simulink model "Variable_spring_CBF_Liu"  (R2023b)
settings: Solver=ode5  StartTime=0.0  StopTime=4  FixedStep=0.0001  RelTol=1e-3
settings Model: Creator=amaiani  LastModifiedBy=amaiani

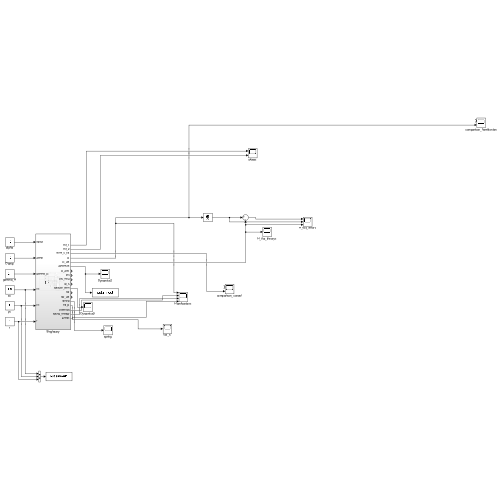
[thumbnail: Simulink's stored preview of the top-level diagram]
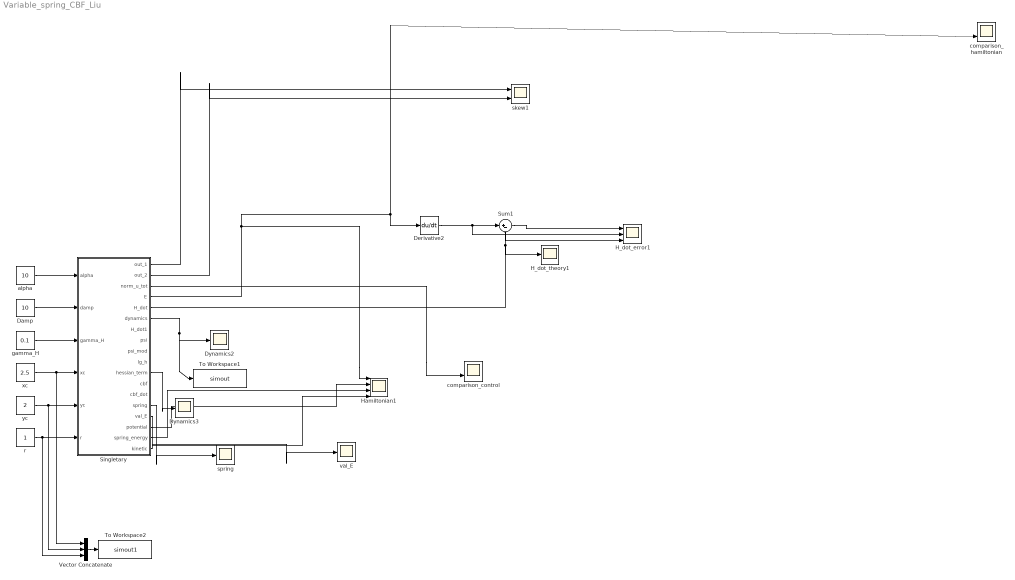
== system Variable_spring_CBF_Liu ==
  Damp : Constant  Value=10
  Derivative2 : Derivative
  Dynamics2 : Scope
  Dynamics3 : Scope
  H_dot_error1 : Scope  NumInputPorts=3
  H_dot_theory1 : Scope
  Hamiltonian1 : Scope  NumInputPorts=4
  Singletary : Subsystem
  Sum1 : Sum  Inputs=|+-
  To Workspace1 : ToWorkspace  VariableName=simout  SampleTime=-1
  To Workspace2 : ToWorkspace  VariableName=simout1  SampleTime=-1
  Vector Concatenate : Concatenate  NumInputs=3
  alpha : Constant  Value=10
  comparison_control : Scope  NumInputPorts=2
  comparison_hamiltonian : Scope  NumInputPorts=2
  gamma_H : Constant  Value=0.1
  r : Constant
  skew1 : Scope  NumInputPorts=2
  spring : Scope
  val_E : Scope
  xc : Constant  Value=2.5
  yc : Constant  Value=2
  wires:
  Derivative2/1 -> H_dot_error1/2, Sum1/1
  Damp/1 -> Singletary/2(damp)
  Sum1/1 -> H_dot_error1/1
  alpha/1 -> Singletary/1(alpha)
  Singletary/5(H_dot) -> H_dot_theory1/1, H_dot_error1/3, Sum1/2
  Singletary/4(E) -> Derivative2/1, comparison_hamiltonian/2, Hamiltonian1/1
  Singletary/1(out_1) -> skew1/1
  Singletary/2(out_2) -> skew1/2
  Singletary/3(norm_u_tot) -> comparison_control/2
  Singletary/6(dynamics) -> Dynamics2/1, To Workspace1/1
  Singletary/11(hessian_term) -> Dynamics3/1
  Singletary/14(spring) -> spring/1
  Singletary/15(val_E) -> val_E/1
  Singletary/18(kinetic) -> Hamiltonian1/4
  Singletary/17(spring_energy) -> Hamiltonian1/3
  Singletary/16(potential) -> Hamiltonian1/2
  gamma_H/1 -> Singletary/3(gamma_H)
  xc/1 -> Vector Concatenate/1, Singletary/4(xc)
  yc/1 -> Vector Concatenate/2, Singletary/5(yc)
  r/1 -> Vector Concatenate/3, Singletary/6(r)
  Vector Concatenate/1 -> To Workspace2/1

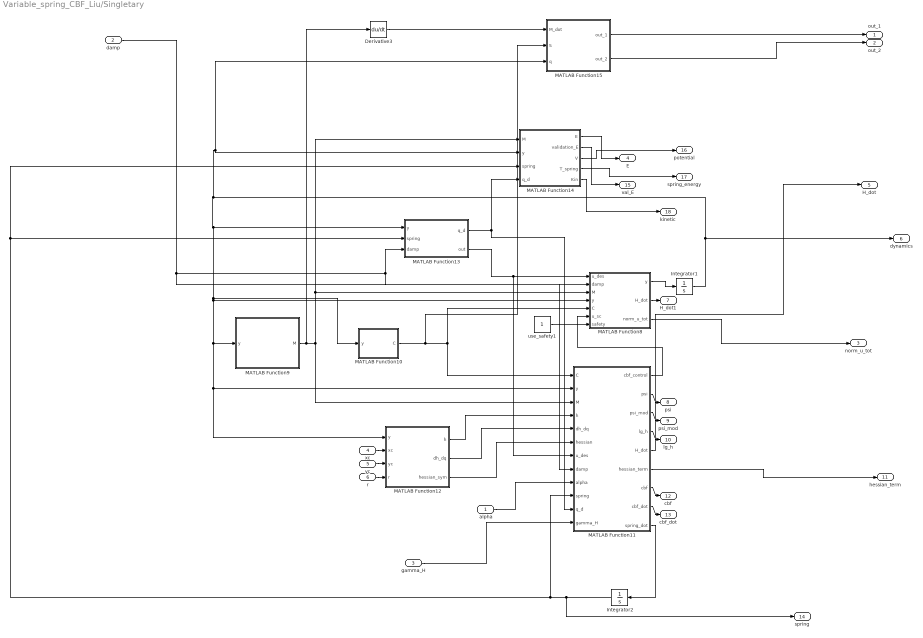
== system Variable_spring_CBF_Liu/Singletary ==
  alpha : Inport
  damp : Inport  Port=2
  gamma_H : Inport  Port=3
  xc : Inport  Port=4
  yc : Inport  Port=5
  r : Inport  Port=6
  Derivative3 : Derivative
  Integrator1 : Integrator  InitialCondition=[0;0;0;0;0;0]
  Integrator2 : Integrator  InitialCondition=[10;10;10]
  MATLAB Function10 : MATLAB Function  StartFcn=|  TreatAsAtomicUnit=on
      | % Define numerical values for the parameters
      | xc = 2.5;
      | yc = 2;
      | r = 1;
      | gamma = 2;
      | alpha = 20;
      | 
      | 
      | m1 = 1;
      | m2 = 1;
      | m3 = 1;
      | 
      | 
      | l1 = 1;
      | l2 = 1;
      | l3 = 1;
  MATLAB Function11 : MATLAB Function  TreatAsAtomicUnit=on
  MATLAB Function12 : MATLAB Function  TreatAsAtomicUnit=on
  MATLAB Function13 : MATLAB Function  TreatAsAtomicUnit=on
  MATLAB Function14 : MATLAB Function  TreatAsAtomicUnit=on
  MATLAB Function15 : MATLAB Function  StartFcn=|  TreatAsAtomicUnit=on
      | % Define numerical values for the parameters
      | xc = 2.5;
      | yc = 2;
      | r = 1;
      | gamma = 2;
      | alpha = 20;
      | 
      | 
      | m1 = 1;
      | m2 = 1;
      | m3 = 1;
      | 
      | 
      | l1 = 1;
      | l2 = 1;
      | l3 = 1;
  MATLAB Function8 : MATLAB Function  TreatAsAtomicUnit=on
  MATLAB Function9 : MATLAB Function  StartFcn=|  TreatAsAtomicUnit=on
      | % Define numerical values for the parameters
      | xc = 2.5;
      | yc = 2;
      | r = 1;
      | gamma = 2;
      | alpha = 20;
      | 
      | 
      | m1 = 1;
      | m2 = 1;
      | m3 = 1;
      | 
      | 
      | l1 = 1;
      | l2 = 1;
      | l3 = 1;
  use_safety1 : Constant
  out_1 : Outport
  out_2 : Outport  Port=2
  norm_u_tot : Outport  Port=3
  E : Outport  Port=4
  H_dot : Outport  Port=5
  dynamics : Outport  Port=6
  H_dot1 : Outport  Port=7
  psi : Outport  Port=8
  psi_mod : Outport  Port=9
  lg_h : Outport  Port=10
  hessian_term : Outport  Port=11
  cbf : Outport  Port=12
  cbf_dot : Outport  Port=13
  spring : Outport  Port=14
  val_E : Outport  Port=15
  potential : Outport  Port=16
  spring_energy : Outport  Port=17
  kinetic : Outport  Port=18
  wires:
  MATLAB Function11/2(psi) -> psi/1
  MATLAB Function11/4(lg_h) -> lg_h/1
  MATLAB Function11/7(cbf) -> cbf/1
  MATLAB Function8/2(H_dot) -> H_dot1/1
  MATLAB Function11/5(H_dot) -> H_dot/1
  MATLAB Function11/6(hessian_term) -> hessian_term/1
  MATLAB Function14/1(E) -> E/1
  MATLAB Function8/3(norm_u_tot) -> norm_u_tot/1
  MATLAB Function12/3(hessian_sym) -> MATLAB Function11/6(hessian)
  Derivative3/1 -> MATLAB Function15/1(M_dot)
  MATLAB Function12/1(h) -> MATLAB Function11/4(h)
  MATLAB Function8/1(y) -> Integrator1/1
  MATLAB Function11/3(psi_mod) -> psi_mod/1
  alpha/1 -> MATLAB Function11/9(alpha)
  MATLAB Function10/1(C) -> MATLAB Function8/5(C), MATLAB Function11/1(C), MATLAB Function15/2(S)
  MATLAB Function11/1(cbf_control) -> MATLAB Function8/6(u_sc)
  MATLAB Function15/2(out_2) -> out_2/1
  Integrator1/1 -> dynamics/1, MATLAB Function15/3(q), MATLAB Function14/2(y), MATLAB Function13/1(y), MATLAB Function10/1(y), MATLAB Function12/1(y), MATLAB Function11/2(y), MATLAB Function9/1(y), MATLAB Function8/4("y ")
  MATLAB Function15/1(out_1) -> out_1/1
  damp/1 -> MATLAB Function11/8(damp), MATLAB Function8/2(damp), MATLAB Function13/3(damp)
  MATLAB Function12/2(dh_dq) -> MATLAB Function11/5(dh_dq)
  MATLAB Function13/2(out) -> MATLAB Function11/7(u_des), MATLAB Function8/1(u_des)
  MATLAB Function11/8(cbf_dot) -> cbf_dot/1
  use_safety1/1 -> MATLAB Function8/7(safety)
  MATLAB Function9/1(M) -> Derivative3/1, MATLAB Function14/1(M), MATLAB Function8/3(M), MATLAB Function11/3(M)
  MATLAB Function11/9(spring_dot) -> Integrator2/1
  Integrator2/1 -> spring/1, MATLAB Function11/10(spring), MATLAB Function13/2(spring), MATLAB Function14/3(spring)
  MATLAB Function13/1(q_d) -> MATLAB Function11/11(q_d), MATLAB Function14/4(q_d)
  MATLAB Function14/2(validation_E) -> val_E/1
  MATLAB Function14/3(V) -> potential/1
  MATLAB Function14/4(T_spring) -> spring_energy/1
  MATLAB Function14/5(Kin) -> kinetic/1
  gamma_H/1 -> MATLAB Function11/12(gamma_H)
  xc/1 -> MATLAB Function12/2(xc)
  yc/1 -> MATLAB Function12/3(yc)
  r/1 -> MATLAB Function12/4(r)

== matlab function Variable_spring_CBF_Liu/Singletary/MATLAB Function8 ==
  data: u_des input; damp input; M input; y input; y output; C input; H_dot output; u_sc input; safety input; norm_u_tot output
function [y,H_dot,norm_u_tot]= dynamics(u_des, damp , M,y, C, u_sc, safety)
    
    q = reshape(y(1:3),[3,1]);
    dq = reshape(y(4:6),[3,1]);



    [~, p] = chol(M);
    decision = (p == 0);

    assert(decision, 'Inertia matrix is not positive definite');
    
    u_tot = u_des + safety * u_sc;
    norm_u_tot=norm(u_tot);
    ddq = inv(M) * (u_tot - C * dq ); % + u_sc

    H_dot = - dq' * damp * dq;

    y = [dq; ddq];

== matlab function Variable_spring_CBF_Liu/Singletary/MATLAB Function9 ==
  data: y input; M output
function M = inertia_M(y)

    q1 = y(1);
    q2 = y(2);
    q3 = y(3);

    M  = [        cos(q2 + q3) + 3*cos(q2) + cos(q3) + 4, cos(q2 + q3)/2 + (3*cos(q2))/2 + cos(q3) + 5/3, cos(q2 + q3)/2 + cos(q3)/2 + 1/3;
cos(q2 + q3)/2 + (3*cos(q2))/2 + cos(q3) + 5/3,                                  cos(q3) + 5/3,                  cos(q3)/2 + 1/3;
              cos(q2 + q3)/2 + cos(q3)/2 + 1/3,                                cos(q3)/2 + 1/3,                              1/3];

== matlab function Variable_spring_CBF_Liu/Singletary/MATLAB Function10 ==
  data: y input; C output
function C = coriolis(y)

    q1 = y(1);
    q2 = y(2);
    q3 = y(3);
    dq1 = y(4);
    dq2 = y(5);
    dq3 = y(6);


    C = [- dq2*(sin(q2 + q3)/2 + (3*sin(q2))/2) - dq3*(sin(q2 + q3)/2 + sin(q3)/2), - dq1*(sin(q2 + q3)/2 + (3*sin(q2))/2) - dq2*(sin(q2 + q3)/2 + (3*sin(q2))/2) - dq3*(sin(q2 + q3)/2 + sin(q3)/2), - dq1*(sin(q2 + q3)/2 + sin(q3)/2) - dq2*(sin(q2 + q3)/2 + sin(q3)/2) - dq3*(sin(q2 + q3)/2 + sin(q3)/2);
                dq1*(sin(q2 + q3)/2 + (3*sin(q2))/2) - (dq3*sin(q3))/2,                                                                                                 -(dq3*sin(q3))/2,                                                    - (dq1*sin(q3))/2 - (dq2*sin(q3))/2 - (dq3*sin(q3))/2;
                       dq1*(sin(q2 + q3)/2 + sin(q3)/2) + (dq2*sin(q3))/2,                                                                                (dq1*sin(q3))/2 + (dq2*sin(q3))/2,                                                                                                        0];

== matlab function Variable_spring_CBF_Liu/Singletary/MATLAB Function11 ==
  data: C input; y input; cbf_control output; M input; h input; dh_dq input; hessian input; u_des input; psi output; psi_mod output; lg_h output; H_dot output; damp input; hessian_term output; cbf output; cbf_dot output; alpha input; spring_dot output; spring input; q_d input; gamma_H input

function [cbf_control, psi, psi_mod,lg_h, H_dot, hessian_term, cbf, cbf_dot, spring_dot]= CBF(C, y, M, h, dh_dq, hessian, u_des, damp, alpha, spring, q_d, gamma_H)
% Define numerical values for the parameters
    xc = 2.5;
    yc = 2;
    r = 1;
    gamma = 2;

    
    m1 = 1;
    m2 = 1;
    m3 = 1;
    
    l1 = 1;
    l2 = 1;
    l3 = 1;
    
    q = reshape(y(1:3),[3,1]);
    dq = reshape(y(4:6),[3,1]);
    dh_dq = reshape(dh_dq,[1,3]);


    cbf = alpha * h + dh_dq * dq;
    lg_h = zeros(1,3);

    M_inv = inv(M);
    cbf_dot_prior = alpha .* dh_dq * dq + dq' * hessian * dq + dh_dq * (M_inv* (-C * dq + u_des));
    psi = cbf_dot_prior + gamma .* cbf;
    if psi<0
        lg_h = dh_dq * M_inv;
        
        cbf_control =  - lg_h' /(lg_h * lg_h')  .* psi;
        active = 1;
    else
        cbf_control = zeros(3,1);

    end
    cbf_dot = alpha .* dh_dq * dq + dq' * hessian * dq + dh_dq * M_inv* (-C * dq + u_des+ cbf_control);
    psi_mod = cbf_dot + gamma .* cbf;

    
    
    dissipated= - dq' * damp * dq;

    hessian_term = dq' * hessian * dq;
    
    spring_dot = zeros(3,1);


    H_dot = dq' * cbf_control - dq' * damp * dq + gamma_H * (0.5 * dq' * M * dq + 0.5 * (q-q_d)' * diag(spring) * (q-q_d) + 0.5 * spring' * spring);
    if psi<0
        error_term = 0.5 * (q-q_d) .* (q-q_d);
        
        A_matrix = error_term' + spring';
    
        spring_dot = -A_matrix'/norm(A_matrix')^2*H_dot;
    
        spring_min = 1;
        gamma_spring = 5;
        spring_dot_min=-gamma_spring * (spring-spring_min);
        spring_dot = max(spring_dot,spring_dot_min);
        spring_dot = min(spring_dot,10 * ones(3,1));
        H_dot = H_dot + A_matrix * spring_dot;
    else

        spring_dot = zeros(3,1);
    end
    
end

== matlab function Variable_spring_CBF_Liu/Singletary/MATLAB Function12 ==
  data: y input; h output; dh_dq output; hessian_sym output; xc input; yc input; r input
function [h, dh_dq, hessian_sym] = obstacle(y,xc,yc,r)
    % Define numerical values for the parameters
    % xc = -2.5;
    % yc = 2;
    % r = 1;

    l1 = 1;
    l2 = 1;
    l3 = 1;
    
    % Compute the end-effector position using forward kinematics
    q1 = y(1);
    q2 = y(2);
    q3 = y(3);
    
    x_ee = l1 * cos(q1) + l2 * cos(q1 + q2) + l3 * cos(q1 + q2 + q3);
    y_ee = l1 * sin(q1) + l2 * sin(q1 + q2) + l3 * sin(q1 + q2 + q3);
    
    % Compute the control barrier function h
    h = (xc - x_ee)^2 + (yc - y_ee)^2 - r^2;
    
    % Define the expressions for dh_dq and hessian_sym
    % dh_dq = [2*(cos(q1 + q2 + q3) + cos(q1 + q2) + cos(q1))*(sin(q1 + q2 + q3) + sin(q1 + q2) + sin(q1) - 2) - 2*(sin(q1 + q2 + q3) + sin(q1 + q2) + sin(q1))*(cos(q1 + q2 + q3) + cos(q1 + q2) + cos(q1) - 5/2), 2*(cos(q1 + q2 + q3) + cos(q1 + q2))*(sin(q1 + q2 + q3) + sin(q1 + q2) + sin(q1) - 2) - 2*(sin(q1 + q2 + q3) + sin(q1 + q2))*(cos(q1 + q2 + q3) + cos(q1 + q2) + cos(q1) - 5/2), 2*cos(q1 + q2 + q3)*(sin(q1 + q2 + q3) + sin(q1 + q2) + sin(q1) - 2) - 2*sin(q1 + q2 + q3)*(cos(q1 + q2 + q3) + cos(q1 + q2) + cos(q1) - 5/2)];
    dh_dq = [2*(cos(q1 + q2 + q3) + cos(q1 + q2) + cos(q1))*(sin(q1 + q2 + q3) - yc + sin(q1 + q2) + sin(q1)) - 2*(sin(q1 + q2 + q3) + sin(q1 + q2) + sin(q1))*(cos(q1 + q2 + q3) - xc + cos(q1 + q2) + cos(q1)), 2*(cos(q1 + q2 + q3) + cos(q1 + q2))*(sin(q1 + q2 + q3) - yc + sin(q1 + q2) + sin(q1)) - 2*(sin(q1 + q2 + q3) + sin(q1 + q2))*(cos(q1 + q2 + q3) - xc + cos(q1 + q2) + cos(q1)), 2*cos(q1 + q2 + q3)*(sin(q1 + q2 + q3) - yc + sin(q1 + q2) + sin(q1)) - 2*sin(q1 + q2 + q3)*(cos(q1 + q2 + q3) - xc + cos(q1 + q2) + cos(q1))];
 

    % hessian_sym = [                                              2*(cos(q1 + q2 + q3) + cos(q1 + q2) + cos(q1))^2 - 2*(cos(q1 + q2 + q3) + cos(q1 + q2) + cos(q1))*(cos(q1 + q2 + q3) + cos(q1 + q2) + cos(q1) - 5/2) + 2*(sin(q1 + q2 + q3) + sin(q1 + q2) + sin(q1))^2 - 2*(sin(q1 + q2 + q3) + sin(q1 + q2) + sin(q1))*(sin(q1 + q2 + q3) + sin(q1 + q2) + sin(q1) - 2), 2*(cos(q1 + q2 + q3) + cos(q1 + q2))*(cos(q1 + q2 + q3) + cos(q1 + q2) + cos(q1)) - 2*(cos(q1 + q2 + q3) + cos(q1 + q2))*(cos(q1 + q2 + q3) + cos(q1 + q2) + cos(q1) - 5/2) + 2*(sin(q1 + q2 + q3) + sin(q1 + q2))*(sin(q1 + q2 + q3) + sin(q1 + q2) + sin(q1)) - 2*(sin(q1 + q2 + q3) + sin(q1 + q2))*(sin(q1 + q2 + q3) + sin(q1 + q2) + sin(q1) - 2), 2*cos(q1 + q2 + q3)*(cos(q1 + q2 + q3) + cos(q1 + q2) + cos(q1)) - 2*cos(q1 + q2 + q3)*(cos(q1 + q2 + q3) + cos(q1 + q2) + cos(q1) - 5/2) + 2*sin(q1 + q2 + q3)*(sin(q1 + q2 + q3) + sin(q1 + q2) + sin(q1)) - 2*sin(q1 + q2 + q3)*(sin(q1 + q2 + q3) + sin(q1 + q2) + sin(q1) - 2);
    %     2*(cos(q1 + q2 + q3) + cos(q1 + q2))*(cos(q1 + q2 + q3) + cos(q1 + q2) + cos(q1)) - 2*(cos(q1 + q2 + q3) + cos(q1 + q2))*(cos(q1 + q2 + q3) + cos(q1 + q2) + cos(q1) - 5/2) + 2*(sin(q1 + q2 + q3) + sin(q1 + q2))*(sin(q1 + q2 + q3) + sin(q1 + q2) + sin(q1)) - 2*(sin(q1 + q2 + q3) + sin(q1 + q2))*(sin(q1 + q2 + q3) + sin(q1 + q2) + sin(q1) - 2),                                                                                       2*(cos(q1 + q2 + q3) + cos(q1 + q2))^2 - 2*(cos(q1 + q2 + q3) + cos(q1 + q2))*(cos(q1 + q2 + q3) + cos(q1 + q2) + cos(q1) - 5/2) + 2*(sin(q1 + q2 + q3) + sin(q1 + q2))^2 - 2*(sin(q1 + q2 + q3) + sin(q1 + q2))*(sin(q1 + q2 + q3) + sin(q1 + q2) + sin(q1) - 2),                     2*cos(q1 + q2 + q3)*(cos(q1 + q2 + q3) + cos(q1 + q2)) - 2*cos(q1 + q2 + q3)*(cos(q1 + q2 + q3) + cos(q1 + q2) + cos(q1) - 5/2) - 2*sin(q1 + q2 + q3)*(sin(q1 + q2 + q3) + sin(q1 + q2) + sin(q1) - 2) + 2*sin(q1 + q2 + q3)*(sin(q1 + q2 + q3) + sin(q1 + q2));
    %                                                                         2*cos(q1 + q2 + q3)*(cos(q1 + q2 + q3) + cos(q1 + q2) + cos(q1)) - 2*cos(q1 + q2 + q3)*(cos(q1 + q2 + q3) + cos(q1 + q2) + cos(q1) - 5/2) + 2*sin(q1 + q2 + q3)*(sin(q1 + q2 + q3) + sin(q1 + q2) + sin(q1)) - 2*sin(q1 + q2 + q3)*(sin(q1 + q2 + q3) + sin(q1 + q2) + sin(q1) - 2),                                                                                         2*cos(q1 + q2 + q3)*(cos(q1 + q2 + q3) + cos(q1 + q2)) - 2*cos(q1 + q2 + q3)*(cos(q1 + q2 + q3) + cos(q1 + q2) + cos(q1) - 5/2) - 2*sin(q1 + q2 + q3)*(sin(q1 + q2 + q3) + sin(q1 + q2) + sin(q1) - 2) + 2*sin(q1 + q2 + q3)*(sin(q1 + q2 + q3) + sin(q1 + q2)),                                                                                       2*cos(q1 + q2 + q3)^2 - 2*cos(q1 + q2 + q3)*(cos(q1 + q2 + q3) + cos(q1 + q2) + cos(q1) - 5/2) + 2*sin(q1 + q2 + q3)^2 - 2*sin(q1 + q2 + q3)*(sin(q1 + q2 + q3) + sin(q1 + q2) + sin(q1) - 2)];
    % 
    % 
    hessian_sym =    [                                              2*(cos(q1 + q2 + q3) + cos(q1 + q2) + cos(q1))^2 - 2*(cos(q1 + q2 + q3) + cos(q1 + q2) + cos(q1))*(cos(q1 + q2 + q3) - xc + cos(q1 + q2) + cos(q1)) - 2*(sin(q1 + q2 + q3) + sin(q1 + q2) + sin(q1))*(sin(q1 + q2 + q3) - yc + sin(q1 + q2) + sin(q1)) + 2*(sin(q1 + q2 + q3) + sin(q1 + q2) + sin(q1))^2, 2*(cos(q1 + q2 + q3) + cos(q1 + q2))*(cos(q1 + q2 + q3) + cos(q1 + q2) + cos(q1)) - 2*(cos(q1 + q2 + q3) + cos(q1 + q2))*(cos(q1 + q2 + q3) - xc + cos(q1 + q2) + cos(q1)) - 2*(sin(q1 + q2 + q3) + sin(q1 + q2))*(sin(q1 + q2 + q3) - yc + sin(q1 + q2) + sin(q1)) + 2*(sin(q1 + q2 + q3) + sin(q1 + q2))*(sin(q1 + q2 + q3) + sin(q1 + q2) + sin(q1)), 2*cos(q1 + q2 + q3)*(cos(q1 + q2 + q3) + cos(q1 + q2) + cos(q1)) - 2*cos(q1 + q2 + q3)*(cos(q1 + q2 + q3) - xc + cos(q1 + q2) + cos(q1)) - 2*sin(q1 + q2 + q3)*(sin(q1 + q2 + q3) - yc + sin(q1 + q2) + sin(q1)) + 2*sin(q1 + q2 + q3)*(sin(q1 + q2 + q3) + sin(q1 + q2) + sin(q1));
        2*(cos(q1 + q2 + q3) + cos(q1 + q2))*(cos(q1 + q2 + q3) + cos(q1 + q2) + cos(q1)) - 2*(cos(q1 + q2 + q3) + cos(q1 + q2))*(cos(q1 + q2 + q3) - xc + cos(q1 + q2) + cos(q1)) - 2*(sin(q1 + q2 + q3) + sin(q1 + q2))*(sin(q1 + q2 + q3) - yc + sin(q1 + q2) + sin(q1)) + 2*(sin(q1 + q2 + q3) + sin(q1 + q2))*(sin(q1 + q2 + q3) + sin(q1 + q2) + sin(q1)),                                                                                       2*(cos(q1 + q2 + q3) + cos(q1 + q2))^2 - 2*(cos(q1 + q2 + q3) + cos(q1 + q2))*(cos(q1 + q2 + q3) - xc + cos(q1 + q2) + cos(q1)) - 2*(sin(q1 + q2 + q3) + sin(q1 + q2))*(sin(q1 + q2 + q3) - yc + sin(q1 + q2) + sin(q1)) + 2*(sin(q1 + q2 + q3) + sin(q1 + q2))^2,                     2*cos(q1 + q2 + q3)*(cos(q1 + q2 + q3) + cos(q1 + q2)) - 2*sin(q1 + q2 + q3)*(sin(q1 + q2 + q3) - yc + sin(q1 + q2) + sin(q1)) - 2*cos(q1 + q2 + q3)*(cos(q1 + q2 + q3) - xc + cos(q1 + q2) + cos(q1)) + 2*sin(q1 + q2 + q3)*(sin(q1 + q2 + q3) + sin(q1 + q2));
                                                                            2*cos(q1 + q2 + q3)*(cos(q1 + q2 + q3) + cos(q1 + q2) + cos(q1)) - 2*cos(q1 + q2 + q3)*(cos(q1 + q2 + q3) - xc + cos(q1 + q2) + cos(q1)) - 2*sin(q1 + q2 + q3)*(sin(q1 + q2 + q3) - yc + sin(q1 + q2) + sin(q1)) + 2*sin(q1 + q2 + q3)*(sin(q1 + q2 + q3) + sin(q1 + q2) + sin(q1)),                                                                                         2*cos(q1 + q2 + q3)*(cos(q1 + q2 + q3) + cos(q1 + q2)) - 2*sin(q1 + q2 + q3)*(sin(q1 + q2 + q3) - yc + sin(q1 + q2) + sin(q1)) - 2*cos(q1 + q2 + q3)*(cos(q1 + q2 + q3) - xc + cos(q1 + q2) + cos(q1)) + 2*sin(q1 + q2 + q3)*(sin(q1 + q2 + q3) + sin(q1 + q2)),                                                                                       2*cos(q1 + q2 + q3)^2 - 2*cos(q1 + q2 + q3)*(cos(q1 + q2 + q3) - xc + cos(q1 + q2) + cos(q1)) - 2*sin(q1 + q2 + q3)*(sin(q1 + q2 + q3) - yc + sin(q1 + q2) + sin(q1)) + 2*sin(q1 + q2 + q3)^2];


    % 
    % d = eig(hessian_sym)
    % isposdef = all(d >= 0);
    % 
    % assert(isposdef, 'error hessian');
end

== matlab function Variable_spring_CBF_Liu/Singletary/MATLAB Function13 ==
  data: q_d output; y input; spring input; out output; damp input
function [q_d, out] = u_des(y, spring, damp)


    q = reshape(y(1:3),[3,1]);
    dq = reshape(y(4:6),[3,1]);

    q_d = [pi; 0; pi/4];
    spring = diag(spring);
    
    out =  - damp * dq - spring * (q-q_d);

== matlab function Variable_spring_CBF_Liu/Singletary/MATLAB Function14 ==
  data: M input; E output; y input; spring input; q_d input; validation_E output; V output; T_spring output; Kin output
function [E,validation_E,V,T_spring,Kin] = energy(M,y,spring, q_d)
    q = y(1:3);
    dq = y(4:6);
    
    spring_mat = diag(spring);
    V = 0.5 *  (q-q_d)' * spring_mat * (q-q_d);
    T_spring = 0.5 * norm(spring)^2;
    Kin =  0.5 * (dq' * M * dq);
    E = Kin +V +T_spring ;
    validation_E = 0.5 * (dq' * M * dq) + (q-q_d)'*(q-q_d);

== matlab function Variable_spring_CBF_Liu/Singletary/MATLAB Function15 ==
  data: M_dot input; out_1 output; S input; q input; out_2 output


function [out_1, out_2] = M_dot_coriolis_check(M_dot,S, q)
    dq = reshape(q(4:6),[3,1]);
    
    q1 = q(1);
    q2 = q(2);
    q3 = q(3);
    dq1 = q(4);
    dq2 = q(5);
    dq3 = q(6);

    check = M_dot - 2 * S;


    out_1 = dq' * check * dq;


    M_dot_formula =   [        - dq2*(sin(q2 + q3) + 3*sin(q2)) - dq3*(sin(q2 + q3) + sin(q3)), - dq3*(sin(q2 + q3)/2 + sin(q3)) - dq2*(sin(q2 + q3)/2 + (3*sin(q2))/2), - (dq2*sin(q2 + q3))/2 - dq3*(sin(q2 + q3)/2 + sin(q3)/2);
- dq3*(sin(q2 + q3)/2 + sin(q3)) - dq2*(sin(q2 + q3)/2 + (3*sin(q2))/2),                                                            -dq3*sin(q3),                                          -(dq3*sin(q3))/2;
              - (dq2*sin(q2 + q3))/2 - dq3*(sin(q2 + q3)/2 + sin(q3)/2),                                                        -(dq3*sin(q3))/2,                                                         0];
 

    
    out_2 = dq' * (M_dot_formula - 2 * S) * dq;
end
